simulink model "inverted_pendulum_SVFB"  (R2020a)
settings: Solver=VariableStepAuto  StartTime=0.0  StopTime=60  RelTol=1e-3
settings Model: Creator=sidsu  LastModifiedBy=sidsu
settings SolverCC: AlgebraicLoopSolver=LineSearch

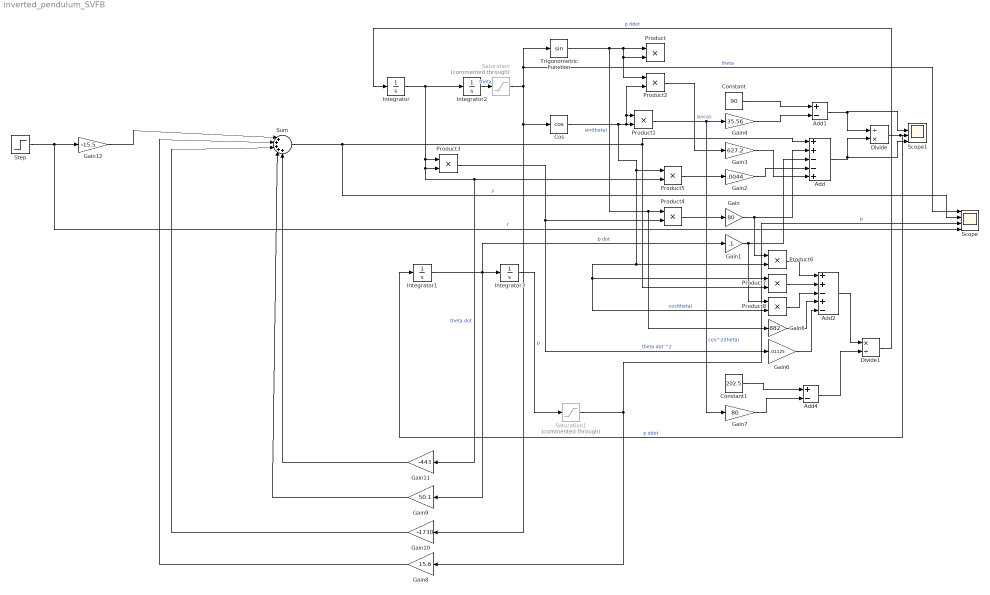
== system inverted_pendulum_SVFB ==
  Add : Sum  Inputs=++--+
  Add1 : Sum  Inputs=+-
  Add2 : Sum  Inputs=++-+-
  Add4 : Sum  Inputs=+-
  Constant : Constant  Value=90
  Constant1 : Constant  Value=202.5
  Cos : Trigonometry  Operator=cos
  Divide : Product  Inputs=/*
  Divide1 : Product  Inputs=*/
  Gain : Gain  Gain=80
  Gain1 : Gain  Gain=.1
  Gain10 : Gain  Gain=-1730
  Gain11 : Gain  Gain=-443
  Gain12 : Gain  Gain=-15.5
  Gain2 : Gain  Gain=.0044
  Gain3 : Gain  Gain=627.2
  Gain4 : Gain  Gain=35.56
  Gain5 : Gain  Gain=882
  Gain6 : Gain  Gain=.01125
  Gain7 : Gain  Gain=80
  Gain8 : Gain  Gain=15.6
  Gain9 : Gain  Gain=50.1
  Integrator{,1..3} (4 alike) : Integrator
  Product{,1..8} (9 alike) : Product
  Saturation : Saturate  Commented=through
  Saturation1 : Saturate  Commented=through  UpperLimit=1  LowerLimit=-1
  Scope : Scope  NumInputPorts=4
  Scope1 : Scope  NumInputPorts=4
  Step : Step  SampleTime=0
  Sum : Sum  Inputs=|+++++
  Trigonometric Function : Trigonometry
  wires:
  Saturation1/1 -> Gain8/1, Scope/3  "p"
  Gain7/1 -> Add4/2
  Add4/1 -> Divide1/2
  Add2/1 -> Divide1/1
  Divide/1 -> Integrator1/1, Scope1/3  "p ddot"
  Product8/1 -> Add2/3
  Product6/1 -> Add2/1
  Gain5/1 -> Add2/4
  Constant1/1 -> Add4/1
  Gain3/1 -> Add/5
  Gain/1 -> Add/2, Product6/1
  Product2/1 -> Gain3/1  "sincos"
  Gain2/1 -> Add/4
  Add/1 -> Scope1/4, Divide/2
  Gain1/1 -> Add/3, Product8/1
  Product3/1 -> Gain6/1, Product4/2  "theta dot ^2"
  Gain4/1 -> Add1/2
  Product5/1 -> Gain2/1
  Product4/1 -> Gain/1
  Saturation/1 -> Gain10/1, Cos/1, Scope/1, Trigonometric Function/1  "theta"
  Integrator1/1 -> Gain9/1, Gain1/1, Integrator3/1  "p dot"
  Integrator/1 -> Integrator2/1, Gain11/1, Product5/2, Product3/2, Product3/1  "theta dot"
  Divide1/1 -> Integrator/1  "p ddot"
  Trigonometric Function/1 -> Gain5/1, Product4/1, Product2/1, Product/2, Product/1  "sin(theta)"
  Product1/1 -> Gain7/1, Gain4/1  "cos^2(theta)"
  Constant/1 -> Add1/1
  Gain6/1 -> Add2/5
  Sum/1 -> Scope/2, Product7/2, Add/1  "F"
  Cos/1 -> Product8/2, Product7/1, Product6/2, Product5/1, Product2/2, Product1/1, Product1/2  "cos(theta)"
  Add1/1 -> Divide/1, Scope1/2
  Product7/1 -> Add2/2
  Gain11/1 -> Sum/5
  Gain9/1 -> Sum/4
  Gain10/1 -> Sum/3
  Gain8/1 -> Sum/2
  Step/1 -> Scope/4, Gain12/1  "r"
  Gain12/1 -> Sum/1
  Integrator2/1 -> Saturation/1  "theta"
  Integrator3/1 -> Saturation1/1  "p"
